simulink model "buckandboost"  (Simulink 7.8)
settings: Solver=ode45  StartTime=0.0  StopTime=0.1  RelTol=1e-3
libraries: powerlib x21, powerlib_extras x3
settings Model: Creator=Administrator  LastModifiedBy=赵
settings DebuggingCC: FcnCallInpInsideContextMsg=Use local settings  StrictBusMsg=Warning

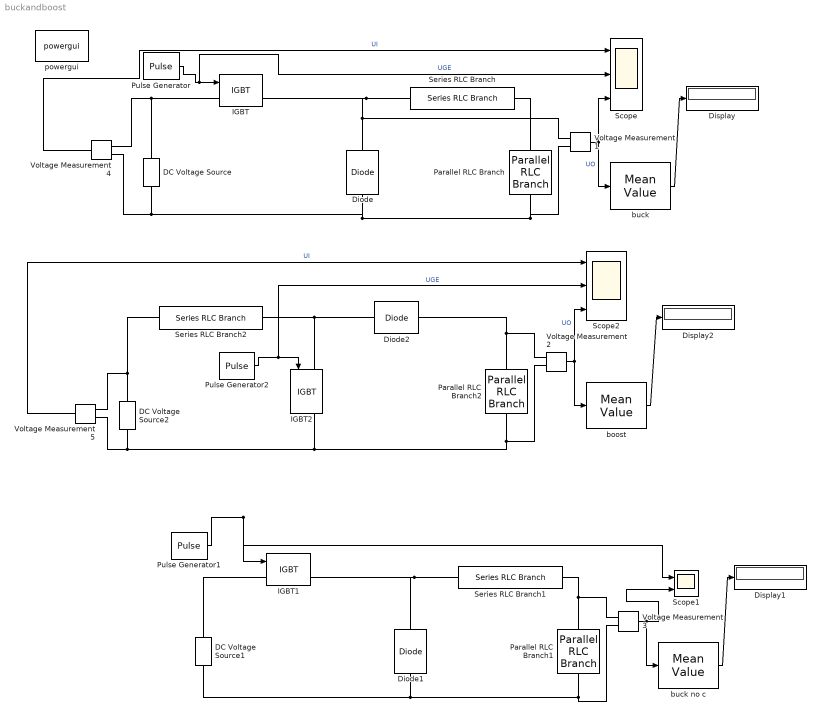
== system buckandboost ==
  DC Voltage Source : powerlib/Electrical Sources/DC Voltage Source  Amplitude=100  Measurements=None
  DC Voltage Source1 : powerlib/Electrical Sources/DC Voltage Source  Amplitude=100  Measurements=None
  DC Voltage Source2 : powerlib/Electrical Sources/DC Voltage Source  Amplitude=100  Measurements=None
  Diode : powerlib/Power Electronics/Diode  Ron=0.001  Lon=0  Vf=0.8  IC=0  UseSnubber=off  Rs=500  Cs=250e-9  Measurements=off
  Diode1 : powerlib/Power Electronics/Diode  Ron=0.001  Lon=0  Vf=0.8  IC=0  UseSnubber=off  Rs=500  Cs=250e-9  Measurements=off
  Diode2 : powerlib/Power Electronics/Diode  Ron=0.001  Lon=0  Vf=0.8  IC=0  UseSnubber=off  Rs=500  Cs=250e-9  Measurements=off
  Display : Display
  Display1 : Display
  Display2 : Display
  IGBT : powerlib/Power Electronics/IGBT  Ron=0.001  Lon=0  Vf=1  Tf=1e-6  Tt=2e-6  IC=0  Rs=1e5  Cs=inf  Measurements=on
  IGBT1 : powerlib/Power Electronics/IGBT  Ron=0.001  Lon=0  Vf=1  Tf=1e-6  Tt=2e-6  IC=0  Rs=1e5  Cs=inf  Measurements=on
  IGBT2 : powerlib/Power Electronics/IGBT  Ron=0.001  Lon=0  Vf=1  Tf=1e-6  Tt=2e-6  IC=0  Rs=1e5  Cs=inf  Measurements=on
  Parallel RLC Branch : powerlib/Elements/Parallel RLC Branch  LConnTagsString=a  RConnTagsString=__new0  BranchType=RC  Resistance=50  Inductance=1e-3  SetiL0=off  InitialCurrent=0  Capacitance=1e-03  Setx0=off  InitialVoltage=0  Measurements=None
  Parallel RLC Branch1 : powerlib/Elements/Parallel RLC Branch  LConnTagsString=a  RConnTagsString=__new0  BranchType=R  Resistance=50  Inductance=1e-3  SetiL0=off  InitialCurrent=0  Capacitance=1000e-06  Setx0=off  InitialVoltage=0  Measurements=None
  Parallel RLC Branch2 : powerlib/Elements/Parallel RLC Branch  LConnTagsString=a  RConnTagsString=__new0  BranchType=RC  Resistance=50  Inductance=1e-3  SetiL0=off  InitialCurrent=0  Capacitance=1e-03  Setx0=off  InitialVoltage=0  Measurements=None
  Pulse Generator : DiscretePulseGenerator  PulseType=Time based  Amplitude=10  Period=0.02  PulseWidth=50
  Pulse Generator1 : DiscretePulseGenerator  PulseType=Time based  Period=0.02  PulseWidth=50
  Pulse Generator2 : DiscretePulseGenerator  PulseType=Time based  Amplitude=10  Period=0.02  PulseWidth=50
  Scope : Scope  NumInputPorts=3
      settings: YMin=0.95~0~-5  YMax=1.05~100~5
  Scope1 : Scope  NumInputPorts=2
      settings: YMin=-5~-5  YMax=5~5
  Scope2 : Scope  NumInputPorts=3
      settings: YMin=-5~-5~-5  YMax=5~5~5  SaveName=ScopeData2
  Series RLC Branch : powerlib/Elements/Series RLC Branch  LConnTagsString=__new0  RConnTagsString=__new0  BranchType=L  Resistance=50  Inductance=1  SetiL0=off  InitialCurrent=0  Capacitance=1e-6  Setx0=off  InitialVoltage=0  Measurements=None
  Series RLC Branch1 : powerlib/Elements/Series RLC Branch  LConnTagsString=__new0  RConnTagsString=__new0  BranchType=L  Resistance=50  Inductance=1  SetiL0=off  InitialCurrent=0  Capacitance=1e-6  Setx0=off  InitialVoltage=0  Measurements=None
  Series RLC Branch2 : powerlib/Elements/Series RLC Branch  LConnTagsString=__new0  RConnTagsString=__new0  BranchType=L  Resistance=50  Inductance=1  SetiL0=off  InitialCurrent=0  Capacitance=1e-6  Setx0=off  InitialVoltage=0  Measurements=None
  Voltage Measurement{1..5} (5 alike) : powerlib/Measurements/Voltage Measurement  PhasorSimulation=off  OutputType=Complex  PSBequivalent=0
  boost : powerlib_extras/Measurements/Mean Value  Period=1/60
  buck : powerlib_extras/Measurements/Mean Value  Period=1/60
  buck no c : powerlib_extras/Measurements/Mean Value  Period=1/60
  powergui : powerlib/powergui  Priority=1  SimulationMode=Continuous  SolverType=Tustin  SampleTime=50e-6  frequency=60  SPID=off  DisableSnubberDevices=off  DisableRonSwitches=off  DisableVfSwitches=off  SwTol=0  Interpol=off  DisplayEquations=off  FunctionMessages=off  frequencyindice=0  Pbase=100e6  ErrMax=1e-4  Iterations=50  UnitsV=kV  UnitsW=MW  echomessages=off  HookPort=off  EnableUseOfTLC=off  x0status=blocks  RestoreLinks=warning  ResistiveCurrentMeasurement=off  Frange=[0:2:500]  Ylog=off  Xlog=on  ShowGrid=off  save=off  variable=ZData  ZoomFFT=on  StartTime=0.0  cycles=1  DisplayStyle=1  fundamental=60  FreqAxis=off  MaxFrequency=1000  frequencyindicesteady=1  RmsSteady=1  display=off  Ts=0  methode=off
  wires:
  Pulse Generator/1 -> IGBT/1, Scope/2  "UGE"
  Voltage Measurement1/1 -> buck/1, Scope/3  "UO"
  buck/1 -> Display/1
  Pulse Generator1/1 -> IGBT1/1, Scope1/1
  buck no c/1 -> Display1/1
  Voltage Measurement3/1 -> Scope1/2, buck no c/1
  Voltage Measurement2/1 -> boost/1, Scope2/3  "UO"
  boost/1 -> Display2/1
  Pulse Generator2/1 -> IGBT2/1, Scope2/2  "UGE"
  Voltage Measurement4/1 -> Scope/1  "UI"
  Voltage Measurement5/1 -> Scope2/1  "UI"
  connections:
  DC Voltage Source/RConn1 -- IGBT/LConn1 -- Voltage Measurement4/LConn1
  Diode/RConn1 -- Series RLC Branch/RConn1 -- IGBT/RConn1 -- Voltage Measurement1/LConn1
  Parallel RLC Branch/RConn1 -- Voltage Measurement1/LConn2 -- Diode/LConn1 -- DC Voltage Source/LConn1 -- Voltage Measurement4/LConn2
  Series RLC Branch/LConn1 -- Parallel RLC Branch/LConn1
  Series RLC Branch1/RConn1 -- IGBT1/RConn1 -- Diode1/RConn1
  Parallel RLC Branch1/RConn1 -- Diode1/LConn1 -- DC Voltage Source1/LConn1 -- Voltage Measurement3/LConn2
  Voltage Measurement3/LConn1 -- Parallel RLC Branch1/LConn1 -- Series RLC Branch1/LConn1
  DC Voltage Source1/RConn1 -- IGBT1/LConn1
  Parallel RLC Branch2/RConn1 -- Voltage Measurement2/LConn2 -- IGBT2/RConn1 -- DC Voltage Source2/LConn1 -- Voltage Measurement5/LConn2
  IGBT2/LConn1 -- Series RLC Branch2/LConn1 -- Diode2/LConn1
  Voltage Measurement2/LConn1 -- Diode2/RConn1 -- Parallel RLC Branch2/LConn1
  DC Voltage Source2/RConn1 -- Series RLC Branch2/RConn1 -- Voltage Measurement5/LConn1
